simulink library "thc"  (R2021b)
settings: Solver=VariableStepAuto  StartTime=0.0  StopTime=10.0  RelTol=1e-3
undefined symbols (not defined in the file or in its folder): ATHC_ChargingPEUEWPReq_X_C, ATHC_ChargingPEUFanReq_X_C, ATHC_CoolingMCUEWPReq_X_C, ATHC_CoolingMCUFanReq_X_C, ATHC_CoolingPEUEWPReq_X_C, ATHC_CoolingPEUFanReq_X_C, ATHC_CoolingTMEWPReq_X_C, ATHC_CoolingTMFanReq_X_C, ENUM_ACCMODE_AFTERRUNNING, ENUM_ACCMODE_CHARGING, ENUM_ACCMODE_COOLING, ENUM_ACCMODE_OFF, ENUM_ACCMODE_SERVICE, ENUM_EWPPEFault_Running, ENUM_MCUFailGrade_NoFault, ENUM_PMMMODE_CHARGE, ENUM_PMMMODE_DRIVE, ENUM_PMMMODE_LVBATCHRG, ENUM_PMMMODE_POWERUP, KDSC_ServiceModeCoolFanReq_pct, KTHC_AfterrunMCUStartTemp_C, KTHC_AfterrunMCUStopTemp_C, KTHC_AfterrunningModeCoolFanReq_pct, KTHC_AfterrunningModeEWPPEReq_rpm, KTHC_AfterrunTMStartTemp_C, KTHC_AfterrunTMStopTemp_C, KTHC_CoolingEWPDisSpdDem_rpm, KTHC_CoolingEWPEnSpdDem_rpm, KTHC_CoolingFanPWMDis_pct, KTHC_CoolingFanPWMEn_pct, KTHC_EWPFaultBypassSwitch_flag, KTHC_EWPPEFaultSpd_rpm, KTHC_LostEWPCoolingFan_pct, KTHC_MCUDerationCoolFanReq_pct, KTHC_MCUDerationEWPPEReq_rpm, KTHC_MCUTempErrCoolFanReq_pct, KTHC_MCUTempErrEWPPEReq_rpm, KTHC_MCUTempError_C, KTHC_PEUDerationCoolFanReq_pct, KTHC_PEUDerationEWPPEReq_rpm, KTHC_PEUDerationTemp_C, KTHC_PEUTempErrCoolFanReq_pct, KTHC_PEUTempErrEWPPEReq_rpm, KTHC_PEUTempError_C, KTHC_ServiceModeCoolFanCMD_flg, KTHC_ServiceModeCoolFanReq_pct, KTHC_ServiceModeEWPPECMD_flg, KTHC_ServiceModeEWPPEReq_rpm, KTHC_ServiceModeON_flg, KTHC_TMTempErrCoolFanReq_pct, KTHC_TMTempErrEWPPEReq_rpm, KTHC_TMTempError_C, MTHC_ChargingPEUEWPReq_Y_rpm, MTHC_ChargingPEUFanReq_Y_pct, MTHC_CoolingMCUEWPReq_Y_rpm, MTHC_CoolingMCUFanReq_Y_pct, MTHC_CoolingPEUEWPReq_Y_rpm, MTHC_CoolingPEUFanReq_Y_pct, MTHC_CoolingTMEWPReq_Y_rpm, MTHC_CoolingTMFanReq_Y_pct ... (+2)
settings Model: Creator=FVT20341  LastModifiedBy=FVT22063

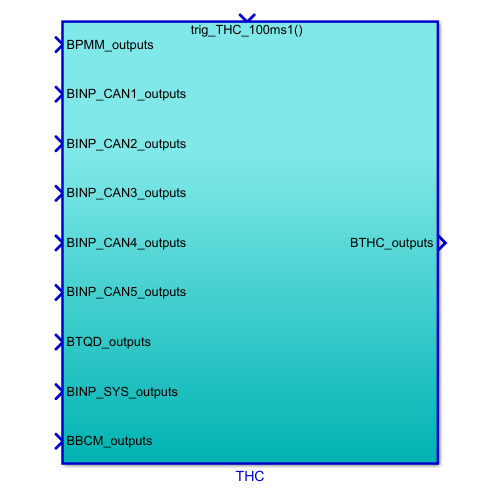
[thumbnail: Simulink's stored preview of the top-level diagram]
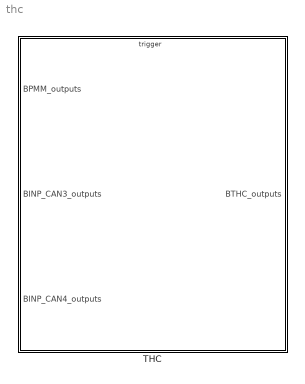
== system thc ==
  THC : Subsystem  TreatAsAtomicUnit=on
      settings: RTWSystemCode=Nonreusable function  RTWFcnNameOpts=Use subsystem name  RTWFileNameOpts=Use subsystem name

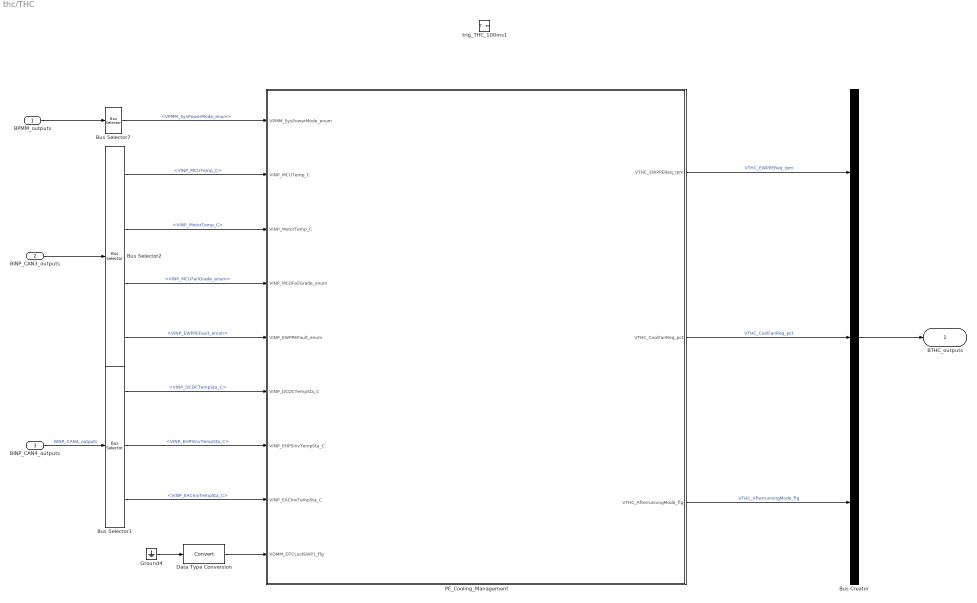
== system thc/THC ==
  BPMM_outputs : Inport  OutDataTypeStr=Bus: BPMM_outputs
  BINP_CAN3_outputs : Inport  Port=2  OutDataTypeStr=Bus: BINP_CAN3_outputs
  BINP_CAN4_outputs : Inport  Port=3  OutDataTypeStr=Bus: BINP_CAN4_outputs
  trig_THC_100ms1 : TriggerPort  TriggerType=function-call  VariantControl=(inherit)
  Bus Creator : BusCreator  Inputs=3  OutDataTypeStr=Bus: BTHC_outputs  NonVirtualBus=on
  Bus Selector1 : BusSelector  OutputSignals=VINP_DCDCTempSta_C,VINP_EHPSInvTempSta_C,VINP_EACInvTempSta_C
  Bus Selector2 : BusSelector  OutputSignals=VINP_MCUTemp_C,VINP_MotorTemp_C,VINP_MCUFailGrade_enum,VINP_EWPPEFault_enum
  Bus Selector7 : BusSelector  OutputSignals=VPMM_SysPowerMode_enum
  Data Type Conversion : DataTypeConversion
  Ground4 : Ground
  PE_Cooling_Management : Subsystem
  BTHC_outputs : Outport  OutDataTypeStr=Bus: BTHC_outputs
  wires:
  BPMM_outputs/1 -> Bus Selector7/1
  BINP_CAN3_outputs/1 -> Bus Selector2/1
  PE_Cooling_Management/1(VTHC_EWPPEReq_rpm) -> Bus Creator/1  "VTHC_EWPPEReq_rpm"
  PE_Cooling_Management/2(VTHC_CoolFanReq_pct) -> Bus Creator/2  "VTHC_CoolFanReq_pct"
  PE_Cooling_Management/3(VTHC_AfterrunningMode_flg) -> Bus Creator/3  "VTHC_AfterrunningMode_flg"
  Bus Creator/1 -> BTHC_outputs/1
  Bus Selector7/1 -> PE_Cooling_Management/1(VPMM_SysPowerMode_enum)  "<VPMM_SysPowerMode_enum>"
  Bus Selector2/1 -> PE_Cooling_Management/2(VINP_MCUTemp_C)  "<VINP_MCUTemp_C>"
  Bus Selector2/2 -> PE_Cooling_Management/3(VINP_MotorTemp_C)  "<VINP_MotorTemp_C>"
  Bus Selector2/3 -> PE_Cooling_Management/4(VINP_MCUFailGrade_enum)  "<VINP_MCUFailGrade_enum>"
  Bus Selector2/4 -> PE_Cooling_Management/5(VINP_EWPPEFault_enum)  "<VINP_EWPPEFault_enum>"
  BINP_CAN4_outputs/1 -> Bus Selector1/1  "BINP_CAN4_outputs"
  Bus Selector1/2 -> PE_Cooling_Management/7(VINP_EHPSInvTempSta_C)  "<VINP_EHPSInvTempSta_C>"
  Bus Selector1/1 -> PE_Cooling_Management/6(VINP_DCDCTempSta_C)  "<VINP_DCDCTempSta_C>"
  Bus Selector1/3 -> PE_Cooling_Management/8(VINP_EACInvTempSta_C)  "<VINP_EACInvTempSta_C>"
  Data Type Conversion/1 -> PE_Cooling_Management/9(VDMM_DTCLostEWP1_flg)
  Ground4/1 -> Data Type Conversion/1

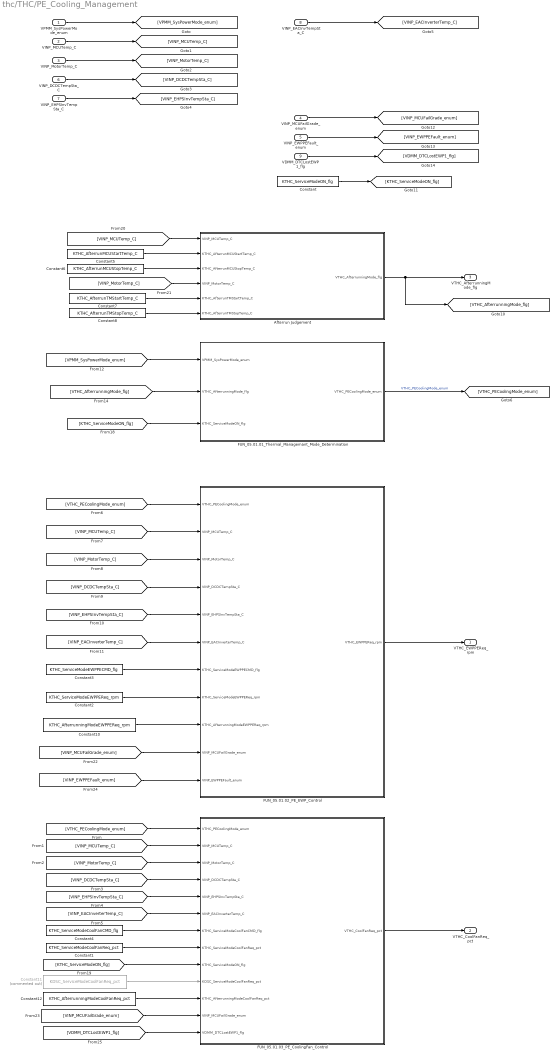
== system thc/THC/PE_Cooling_Management ==
  VPMM_SysPowerMode_enum : Inport
  VINP_MCUTemp_C : Inport  Port=2
  VINP_MotorTemp_C : Inport  Port=3
  VINP_MCUFailGrade_enum : Inport  Port=4
  VINP_EWPPEFault_enum : Inport  Port=5
  VINP_DCDCTempSta_C : Inport  Port=6
  VINP_EHPSInvTempSta_C : Inport  Port=7
  VINP_EACInvTempSta_C : Inport  Port=8
  VDMM_DTCLostEWP1_flg : Inport  Port=9
  Afterrun Judgement : Subsystem
  Constant : Constant  Value=KTHC_ServiceModeON_flg
  Constant1 : Constant  Value=KTHC_ServiceModeCoolFanReq_pct
  Constant10 : Constant  Value=KTHC_AfterrunningModeEWPPEReq_rpm
  Constant11 : Constant  Commented=on  Value=KDSC_ServiceModeCoolFanReq_pct
  Constant12 : Constant  Value=KTHC_AfterrunningModeCoolFanReq_pct
  Constant2 : Constant  Value=KTHC_ServiceModeEWPPEReq_rpm
  Constant3 : Constant  Value=KTHC_ServiceModeEWPPECMD_flg
  Constant4 : Constant  Value=KTHC_ServiceModeCoolFanCMD_flg
  Constant5 : Constant  Value=KTHC_AfterrunMCUStartTemp_C
  Constant6 : Constant  Value=KTHC_AfterrunMCUStopTemp_C
  Constant7 : Constant  Value=KTHC_AfterrunTMStartTemp_C
  Constant8 : Constant  Value=KTHC_AfterrunTMStopTemp_C
  FUN_05.01.01_Thermal_Managemant_Mode_Determination : Subsystem
  FUN_05.01.02_PE_EWP_Control : Subsystem
  FUN_05.01.03_PE_CoolingFan_Control : Subsystem
  VTHC_EWPPEReq_rpm : Outport
  VTHC_CoolFanReq_pct : Outport  Port=2
  VTHC_AfterrunningMode_flg : Outport  Port=3
  wires:
  [VTHC_AfterrunningMode_flg] -> FUN_05.01.01_Thermal_Managemant_Mode_Determination/2(VTHC_AfterrunningMode_flg)
  Constant2/1 -> FUN_05.01.02_PE_EWP_Control/8(KTHC_ServiceModeEWPPEReq_rpm)
  Constant3/1 -> FUN_05.01.02_PE_EWP_Control/7(KTHC_ServiceModeEWPPECMD_flg)
  [VINP_EACInverterTemp_C] -> FUN_05.01.02_PE_EWP_Control/6(VINP_EACInverterTemp_C)
  [VINP_EHPSInvTempSta_C] -> FUN_05.01.02_PE_EWP_Control/5(VINP_EHPSInvTempSta_C)
  [VINP_DCDCTempSta_C] -> FUN_05.01.02_PE_EWP_Control/4(VINP_DCDCTempSta_C)
  [VINP_MotorTemp_C] -> FUN_05.01.02_PE_EWP_Control/3(VINP_MotorTemp_C)
  [VINP_MCUTemp_C] -> FUN_05.01.02_PE_EWP_Control/2(VINP_MCUTemp_C)
  [VTHC_PECoolingMode_enum] -> FUN_05.01.02_PE_EWP_Control/1(VTHC_PECoolingMode_enum)
  Constant1/1 -> FUN_05.01.03_PE_CoolingFan_Control/8(KTHC_ServiceModeCoolFanReq_pct)
  Constant4/1 -> FUN_05.01.03_PE_CoolingFan_Control/7(KTHC_ServiceModeCoolFanCMD_flg)
  [VINP_EACInverterTemp_C] -> FUN_05.01.03_PE_CoolingFan_Control/6(VINP_EACInverterTemp_C)
  [VINP_EHPSInvTempSta_C] -> FUN_05.01.03_PE_CoolingFan_Control/5(VINP_EHPSInvTempSta_C)
  [VINP_DCDCTempSta_C] -> FUN_05.01.03_PE_CoolingFan_Control/4(VINP_DCDCTempSta_C)
  [VINP_MotorTemp_C] -> FUN_05.01.03_PE_CoolingFan_Control/3(VINP_MotorTemp_C)
  [VINP_MCUTemp_C] -> FUN_05.01.03_PE_CoolingFan_Control/2(VINP_MCUTemp_C)
  [VTHC_PECoolingMode_enum] -> FUN_05.01.03_PE_CoolingFan_Control/1(VTHC_PECoolingMode_enum)
  FUN_05.01.02_PE_EWP_Control/1(VTHC_EWPPEReq_rpm) -> VTHC_EWPPEReq_rpm/1
  FUN_05.01.03_PE_CoolingFan_Control/1(VTHC_CoolFanReq_pct) -> VTHC_CoolFanReq_pct/1
  [VPMM_SysPowerMode_enum] -> FUN_05.01.01_Thermal_Managemant_Mode_Determination/1(VPMM_SysPowerMode_enum)
  FUN_05.01.01_Thermal_Managemant_Mode_Determination/1(VTHC_PECoolingMode_enum) -> [VTHC_PECoolingMode_enum]  "VTHC_PECoolingMode_enum"
  VINP_MCUTemp_C/1 -> [VINP_MCUTemp_C]
  VINP_MotorTemp_C/1 -> [VINP_MotorTemp_C]
  VINP_DCDCTempSta_C/1 -> [VINP_DCDCTempSta_C]
  VINP_EHPSInvTempSta_C/1 -> [VINP_EHPSInvTempSta_C]
  VINP_EACInvTempSta_C/1 -> [VINP_EACInverterTemp_C]
  VPMM_SysPowerMode_enum/1 -> [VPMM_SysPowerMode_enum]
  Constant/1 -> [KTHC_ServiceModeON_flg]
  [KTHC_ServiceModeON_flg] -> FUN_05.01.01_Thermal_Managemant_Mode_Determination/3(KTHC_ServiceModeON_flg)
  [KTHC_ServiceModeON_flg] -> FUN_05.01.03_PE_CoolingFan_Control/9(KTHC_ServiceModeON_flg)
  Afterrun Judgement/1(VTHC_AfterrunningMode_flg) -> VTHC_AfterrunningMode_flg/1, [VTHC_AfterrunningMode_flg]
  [VINP_MotorTemp_C] -> Afterrun Judgement/4(VINP_MotorTemp_C)
  [VINP_MCUTemp_C] -> Afterrun Judgement/1(VINP_MCUTemp_C)
  Constant5/1 -> Afterrun Judgement/2(KTHC_AfterrunMCUStartTemp_C)
  Constant6/1 -> Afterrun Judgement/3(KTHC_AfterrunMCUStopTemp_C)
  Constant7/1 -> Afterrun Judgement/5(KTHC_AfterrunTMStartTemp_C)
  Constant8/1 -> Afterrun Judgement/6(KTHC_AfterrunTMStopTemp_C)
  Constant10/1 -> FUN_05.01.02_PE_EWP_Control/9(KTHC_AfterrunningModeEWPPEReq_rpm)
  Constant11/1 -> FUN_05.01.03_PE_CoolingFan_Control/10(KDSC_ServiceModeCoolFanReq_pct)
  Constant12/1 -> FUN_05.01.03_PE_CoolingFan_Control/11(KTHC_AfterrunningModeCoolFanReq_pct)
  VINP_MCUFailGrade_enum/1 -> [VINP_MCUFailGrade_enum]
  [VINP_MCUFailGrade_enum] -> FUN_05.01.02_PE_EWP_Control/10(VINP_MCUFailGrade_enum)
  [VINP_MCUFailGrade_enum] -> FUN_05.01.03_PE_CoolingFan_Control/12(VINP_MCUFailGrade_enum)
  VINP_EWPPEFault_enum/1 -> [VINP_EWPPEFault_enum]
  [VINP_EWPPEFault_enum] -> FUN_05.01.02_PE_EWP_Control/11(VINP_EWPPEFault_enum)
  VDMM_DTCLostEWP1_flg/1 -> [VDMM_DTCLostEWP1_flg]
  [VDMM_DTCLostEWP1_flg] -> FUN_05.01.03_PE_CoolingFan_Control/13(VDMM_DTCLostEWP1_flg)

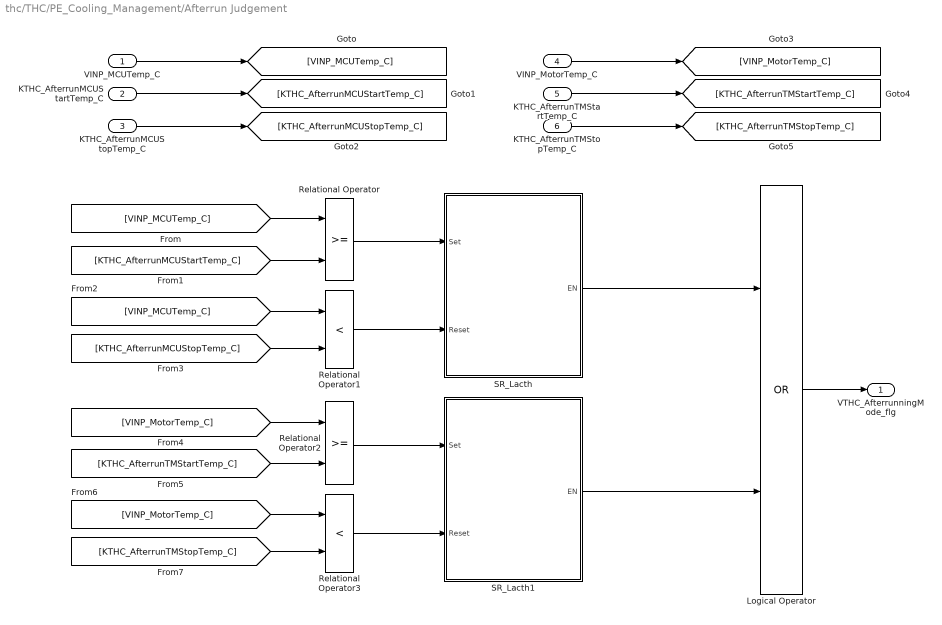
== system thc/THC/PE_Cooling_Management/Afterrun Judgement ==
  VINP_MCUTemp_C : Inport
  KTHC_AfterrunMCUStartTemp_C : Inport  Port=2
  KTHC_AfterrunMCUStopTemp_C : Inport  Port=3
  VINP_MotorTemp_C : Inport  Port=4
  KTHC_AfterrunTMStartTemp_C : Inport  Port=5
  KTHC_AfterrunTMStopTemp_C : Inport  Port=6
  Logical Operator : Logic  Operator=OR  AllPortsSameDT=off  OutDataTypeStr=boolean
  Relational Operator : RelationalOperator  OutDataTypeStr=boolean  RndMeth=Simplest
  Relational Operator1 : RelationalOperator  Operator=<  OutDataTypeStr=boolean  RndMeth=Simplest
  Relational Operator2 : RelationalOperator  OutDataTypeStr=boolean  RndMeth=Simplest
  Relational Operator3 : RelationalOperator  Operator=<  OutDataTypeStr=boolean  RndMeth=Simplest
  SR_Lacth : Subsystem
  SR_Lacth1 : Subsystem
  VTHC_AfterrunningMode_flg : Outport
  wires:
  SR_Lacth/1(EN) -> Logical Operator/1
  VINP_MCUTemp_C/1 -> [VINP_MCUTemp_C]
  KTHC_AfterrunMCUStartTemp_C/1 -> [KTHC_AfterrunMCUStartTemp_C]
  KTHC_AfterrunMCUStopTemp_C/1 -> [KTHC_AfterrunMCUStopTemp_C]
  VINP_MotorTemp_C/1 -> [VINP_MotorTemp_C]
  KTHC_AfterrunTMStartTemp_C/1 -> [KTHC_AfterrunTMStartTemp_C]
  KTHC_AfterrunTMStopTemp_C/1 -> [KTHC_AfterrunTMStopTemp_C]
  [VINP_MCUTemp_C] -> Relational Operator/1
  [KTHC_AfterrunMCUStartTemp_C] -> Relational Operator/2
  Relational Operator/1 -> SR_Lacth/1(Set)
  [KTHC_AfterrunMCUStopTemp_C] -> Relational Operator1/2
  [VINP_MCUTemp_C] -> Relational Operator1/1
  Relational Operator1/1 -> SR_Lacth/2(Reset)
  [KTHC_AfterrunTMStopTemp_C] -> Relational Operator3/2
  [VINP_MotorTemp_C] -> Relational Operator2/1
  SR_Lacth1/1(EN) -> Logical Operator/2
  [KTHC_AfterrunTMStartTemp_C] -> Relational Operator2/2
  Relational Operator3/1 -> SR_Lacth1/2(Reset)
  [VINP_MotorTemp_C] -> Relational Operator3/1
  Logical Operator/1 -> VTHC_AfterrunningMode_flg/1
  Relational Operator2/1 -> SR_Lacth1/1(Set)

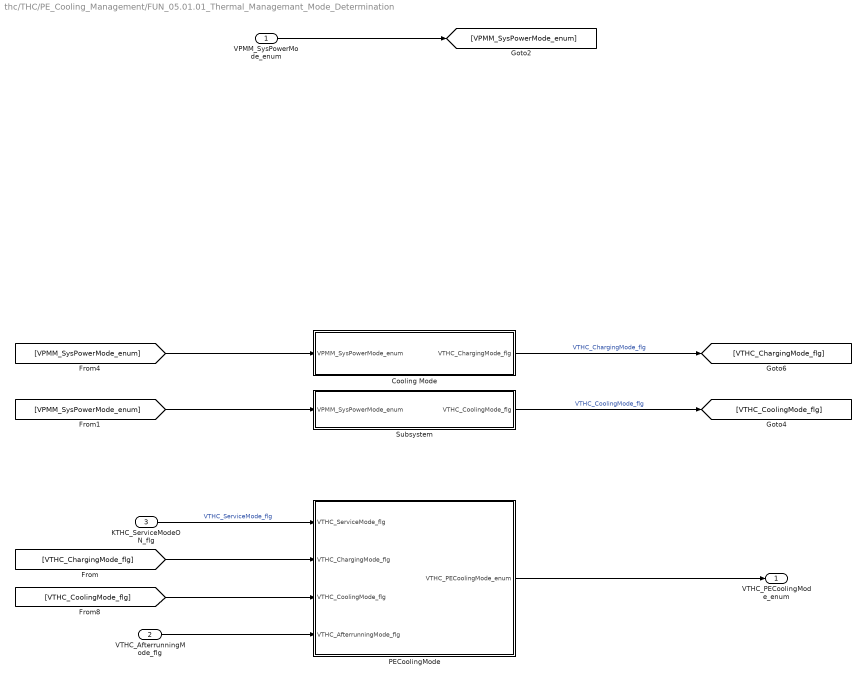
== system thc/THC/PE_Cooling_Management/FUN_05.01.01_Thermal_Managemant_Mode_Determination ==
  VPMM_SysPowerMode_enum : Inport
  VTHC_AfterrunningMode_flg : Inport  Port=2
  KTHC_ServiceModeON_flg : Inport  Port=3
  Cooling Mode : Subsystem
  PECoolingMode : Subsystem
  Subsystem : Subsystem
  VTHC_PECoolingMode_enum : Outport  VectorParamsAs1DForOutWhenUnconnected=off
  wires:
  VTHC_AfterrunningMode_flg/1 -> PECoolingMode/4(VTHC_AfterrunningMode_flg)
  [VTHC_CoolingMode_flg] -> PECoolingMode/3(VTHC_CoolingMode_flg)
  [VTHC_ChargingMode_flg] -> PECoolingMode/2(VTHC_ChargingMode_flg)
  KTHC_ServiceModeON_flg/1 -> PECoolingMode/1(VTHC_ServiceMode_flg)  "VTHC_ServiceMode_flg"
  [VPMM_SysPowerMode_enum] -> Subsystem/1(VPMM_SysPowerMode_enum)
  Subsystem/1(VTHC_CoolingMode_flg) -> [VTHC_CoolingMode_flg]  "VTHC_CoolingMode_flg"
  PECoolingMode/1(VTHC_PECoolingMode_enum) -> VTHC_PECoolingMode_enum/1
  [VPMM_SysPowerMode_enum] -> Cooling Mode/1(VPMM_SysPowerMode_enum)
  VPMM_SysPowerMode_enum/1 -> [VPMM_SysPowerMode_enum]
  Cooling Mode/1(VTHC_ChargingMode_flg) -> [VTHC_ChargingMode_flg]  "VTHC_ChargingMode_flg"

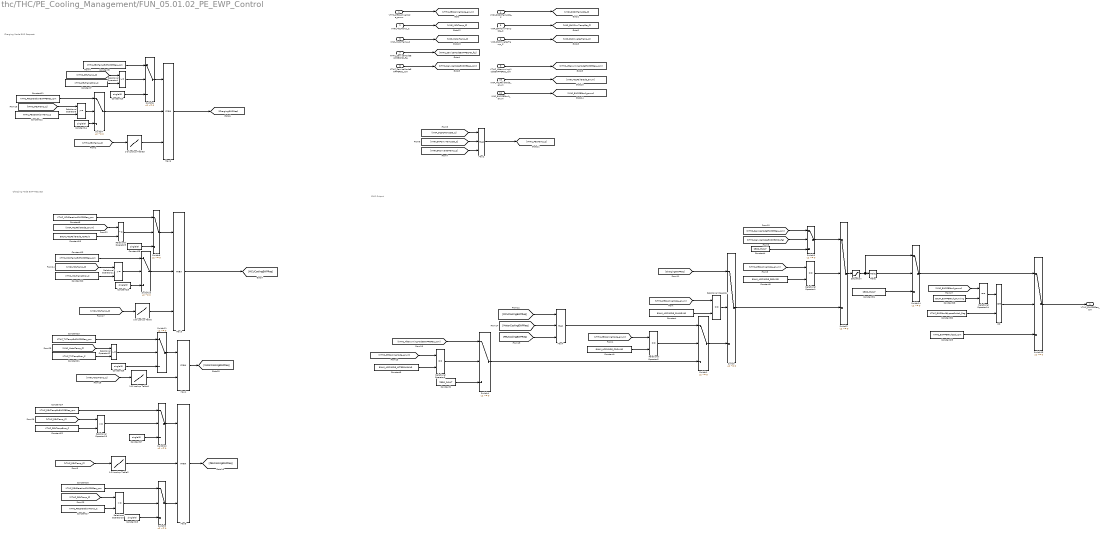
== system thc/THC/PE_Cooling_Management/FUN_05.01.02_PE_EWP_Control ==
  note: EWP Output
  note: Charging Mode EWP Request
  note: Charging Mode EWP Request
  VTHC_PECoolingMode_enum : Inport
  VINP_MCUTemp_C : Inport  Port=2
  VINP_MotorTemp_C : Inport  Port=3
  VINP_DCDCTempSta_C : Inport  Port=4
  VINP_EHPSInvTempSta_C : Inport  Port=5
  VINP_EACInverterTemp_C : Inport  Port=6
  KTHC_ServiceModeEWPPECMD_flg : Inport  Port=7
  KTHC_ServiceModeEWPPEReq_rpm : Inport  Port=8
  KTHC_AfterrunningModeEWPPEReq_rpm : Inport  Port=9
  VINP_MCUFailGrade_enum : Inport  Port=10
  VINP_EWPPEFault_enum : Inport  Port=11
  1-D Lookup Table : Lookup_n-D  NumberOfTableDimensions=1  BreakpointsForDimension1=ATHC_CoolingMCUEWPReq_X_C  Table=MTHC_CoolingMCUEWPReq_Y_rpm  ExtrapMethod=Clip  UseLastTableValue=on  InternalRulePriority=Speed  RndMeth=Simplest  InputSameDT=on
  1-D Lookup Table1 : Lookup_n-D  NumberOfTableDimensions=1  BreakpointsForDimension1=ATHC_CoolingTMEWPReq_X_C  Table=MTHC_CoolingTMEWPReq_Y_rpm  ExtrapMethod=Clip  UseLastTableValue=on  InternalRulePriority=Speed  RndMeth=Simplest  InputSameDT=on
  1-D Lookup Table2 : Lookup_n-D  NumberOfTableDimensions=1  BreakpointsForDimension1=ATHC_CoolingPEUEWPReq_X_C  Table=MTHC_CoolingPEUEWPReq_Y_rpm  ExtrapMethod=Clip  UseLastTableValue=on  InternalRulePriority=Speed  RndMeth=Simplest  InputSameDT=on
  1-D Lookup Table3 : Lookup_n-D  NumberOfTableDimensions=1  BreakpointsForDimension1=ATHC_ChargingPEUEWPReq_X_C  Table=MTHC_ChargingPEUEWPReq_Y_rpm  ExtrapMethod=Clip  UseLastTableValue=on  InternalRulePriority=Speed  RndMeth=Simplest  InputSameDT=on
  Constant : Constant  Value=ENUM_ACCMODE_CHARGING
  Constant1 : Constant  Value=ENUM_ACCMODE_COOLING
  Constant{10,14,18..19,25..27} (7 alike) : Constant  Value=single(0)
  Constant11 : Constant  Value=KTHC_PEUDerationEWPPEReq_rpm
  Constant12 : Constant  Value=KTHC_PEUDerationTemp_C
  Constant13 : Constant  Value=KTHC_MCUTempErrEWPPEReq_rpm
  Constant15 : Constant  Value=ENUM_MCUFailGrade_NoFault
  Constant16 : Constant  Value=KTHC_PEUDerationEWPPEReq_rpm
  Constant17 : Constant  Value=KTHC_PEUDerationTemp_C
  Constant2 : Constant  Value=ZERO_FLOAT
  Constant20 : Constant  Value=KTHC_MCUTempError_C
  Constant21 : Constant  Value=KTHC_TMTempError_C
  Constant22 : Constant  Value=KTHC_PEUTempError_C
  Constant23 : Constant  Value=KTHC_TMTempErrEWPPEReq_rpm
  Constant24 : Constant  Value=KTHC_PEUTempErrEWPPEReq_rpm
  Constant28 : Constant  Value=ENUM_EWPPEFault_Running
  Constant29 : Constant  Value=KTHC_EWPPEFaultSpd_rpm
  Constant3 : Constant  Value=ENUM_ACCMODE_SERVICE
  Constant30 : Constant  Value=KTHC_EWPFaultBypassSwitch_flag  VectorParams1D=off
  Constant31 : Constant  Value=ZERO_FLOAT
  Constant4 : Constant  Value=ZERO_FLOAT
  Constant5 : Constant  Value=ENUM_ACCMODE_AFTERRUNNING
  Constant7 : Constant  Value=KTHC_PEUTempError_C
  Constant8 : Constant  Value=KTHC_MCUDerationEWPPEReq_rpm
  Constant9 : Constant  Value=KTHC_PEUTempErrEWPPEReq_rpm
  Max1 : MinMax  Function=max  Inputs=2
  Max{2..6} (5 alike) : MinMax  Function=max  Inputs=3
  OR : Logic  Operator=OR  AllPortsSameDT=off  OutDataTypeStr=boolean
  Relational Operator{,1..3,14} (5 alike) : RelationalOperator  Operator===  OutDataTypeStr=boolean  RndMeth=Simplest
  Relational Operator{4..5,10..13} (6 alike) : RelationalOperator  OutDataTypeStr=boolean  RndMeth=Simplest
  Relational Operator9 : RelationalOperator  Operator=~=  OutDataTypeStr=boolean  RndMeth=Simplest
  Relay : Relay  OnSwitchValue=KTHC_CoolingEWPEnSpdDem_rpm  OffSwitchValue=KTHC_CoolingEWPDisSpdDem_rpm  OnOutputValue=TRUE  OffOutputValue=FALSE  OutDataTypeStr=boolean
  Saturation : Saturate  UpperLimit=6000  LowerLimit=0
  Switch{,1..4,6..14} (14 alike) : Switch  Criteria=u2 ~= 0
  VTHC_EWPPEReq_rpm : Outport
  wires:
  VINP_MCUTemp_C/1 -> [VINP_MCUTemp_C]
  Switch2/1 -> Saturation/1
  [KTHC_AfterrunningModeEWPPEReq_rpm] -> Switch4/1
  Constant2/1 -> Switch4/3
  [VTHC_PECoolingMode_enum] -> Relational Operator3/1
  Relational Operator3/1 -> Switch4/2
  Constant5/1 -> Relational Operator3/2
  Switch4/1 -> Switch1/3
  KTHC_ServiceModeEWPPEReq_rpm/1 -> [KTHC_ServiceModeEWPPEReq_rpm]
  KTHC_ServiceModeEWPPECMD_flg/1 -> [KTHC_ServiceModeEWPPECMD_flg]
  VINP_MotorTemp_C/1 -> [VINP_MotorTemp_C]
  VTHC_PECoolingMode_enum/1 -> [VTHC_PECoolingMode_enum]
  [VTHC_PECoolingMode_enum] -> Relational Operator/1
  [VTHC_PECoolingMode_enum] -> Relational Operator2/1
  [VINP_EACInverterTemp_C] -> Max2/3
  [VINP_DCDCTempSta_C] -> Max2/1
  [VINP_EHPSInvTempSta_C] -> Max2/2
  Relational Operator/1 -> Switch/2
  Max2/1 -> [VTHC_PEUTemp_C]
  [VTHC_PEUTemp_C] -> 1-D Lookup Table2/1
  Constant1/1 -> Relational Operator2/2
  [KTHC_ServiceModeEWPPECMD_flg] -> Switch3/2
  Switch/1 -> Switch2/3
  Constant/1 -> Relational Operator/2
  Switch1/1 -> Switch/3
  Relational Operator2/1 -> Switch1/2
  Relational Operator1/1 -> Switch2/2
  Constant4/1 -> Switch3/3
  [VTHC_PECoolingMode_enum] -> Relational Operator1/1
  Constant3/1 -> Relational Operator1/2
  [KTHC_ServiceModeEWPPEReq_rpm] -> Switch3/1
  VINP_DCDCTempSta_C/1 -> [VINP_DCDCTempSta_C]
  VINP_EHPSInvTempSta_C/1 -> [VINP_EHPSInvTempSta_C]
  VINP_EACInverterTemp_C/1 -> [VINP_EACInverterTemp_C]
  Switch3/1 -> Switch2/1
  KTHC_AfterrunningModeEWPPEReq_rpm/1 -> [KTHC_AfterrunningModeEWPPEReq_rpm]
  VINP_MCUFailGrade_enum/1 -> [VINP_MCUFailGrade_enum]
  [VTHC_PEUTemp_C] -> 1-D Lookup Table3/1
  [VINP_MCUTemp_C] -> 1-D Lookup Table/1
  [VINP_MotorTemp_C] -> 1-D Lookup Table1/1
  [VINP_MCUFailGrade_enum] -> Relational Operator9/1
  Relational Operator9/1 -> Switch8/2
  Constant15/1 -> Relational Operator9/2
  Constant16/1 -> Switch9/1
  Constant17/1 -> Relational Operator10/2
  Relational Operator10/1 -> Switch9/2
  [VTHC_PEUTemp_C] -> Relational Operator10/1
  Constant8/1 -> Switch8/1
  Constant18/1 -> Switch8/3
  Constant19/1 -> Switch9/3
  Constant20/1 -> Relational Operator11/2
  Constant22/1 -> Relational Operator13/2
  [VINP_MCUTemp_C] -> Relational Operator11/1
  [VINP_MotorTemp_C] -> Relational Operator12/1
  [VTHC_PEUTemp_C] -> Relational Operator13/1
  Constant21/1 -> Relational Operator12/2
  Relational Operator11/1 -> Switch10/2
  Relational Operator12/1 -> Switch11/2
  Relational Operator13/1 -> Switch12/2
  Constant25/1 -> Switch10/3
  Constant26/1 -> Switch11/3
  Constant27/1 -> Switch12/3
  Constant24/1 -> Switch12/1
  Constant23/1 -> Switch11/1
  Constant13/1 -> Switch10/1
  VINP_EWPPEFault_enum/1 -> [VINP_EWPPEFault_enum]
  [VINP_EWPPEFault_enum] -> Relational Operator14/1
  Constant28/1 -> Relational Operator14/2
  Switch13/1 -> VTHC_EWPPEReq_rpm/1
  Constant29/1 -> Switch13/3
  Switch10/1 -> Max3/2
  1-D Lookup Table/1 -> Max3/3
  Switch8/1 -> Max3/1
  Switch11/1 -> Max1/1
  1-D Lookup Table1/1 -> Max1/2
  Switch12/1 -> Max5/1
  1-D Lookup Table2/1 -> Max5/2
  Switch9/1 -> Max5/3
  Max3/1 -> [MCUCoolingEWPReq]
  [VTHC_PEUTemp_C] -> Relational Operator4/1
  Relational Operator4/1 -> Switch6/2
  Constant12/1 -> Relational Operator5/2
  Constant9/1 -> Switch6/1
  Constant7/1 -> Relational Operator4/2
  Constant11/1 -> Switch7/1
  Relational Operator5/1 -> Switch7/2
  Constant10/1 -> Switch6/3
  [VTHC_PEUTemp_C] -> Relational Operator5/1
  Constant14/1 -> Switch7/3
  Switch6/1 -> Max6/1
  Switch7/1 -> Max6/2
  1-D Lookup Table3/1 -> Max6/3
  Max6/1 -> [ChargingEWPReq]
  Relational Operator14/1 -> OR/1
  Saturation/1 -> Relay/1, Switch14/1  "VTHC_OriginalEWPSpdDem_rpm"
  Relay/1 -> Switch14/2  "VTHC_EWPSpdDemRelay_flg"
  Switch14/1 -> Switch13/1
  Constant31/1 -> Switch14/3
  Constant30/1 -> OR/2
  OR/1 -> Switch13/2
  [ChargingEWPReq] -> Switch/1
  Max1/1 -> [MotorCoolingEWPReq]
  Max5/1 -> [PEUCoolingEWPReq]
  Max4/1 -> Switch1/1
  [MCUCoolingEWPReq] -> Max4/1
  [MotorCoolingEWPReq] -> Max4/2
  [PEUCoolingEWPReq] -> Max4/3

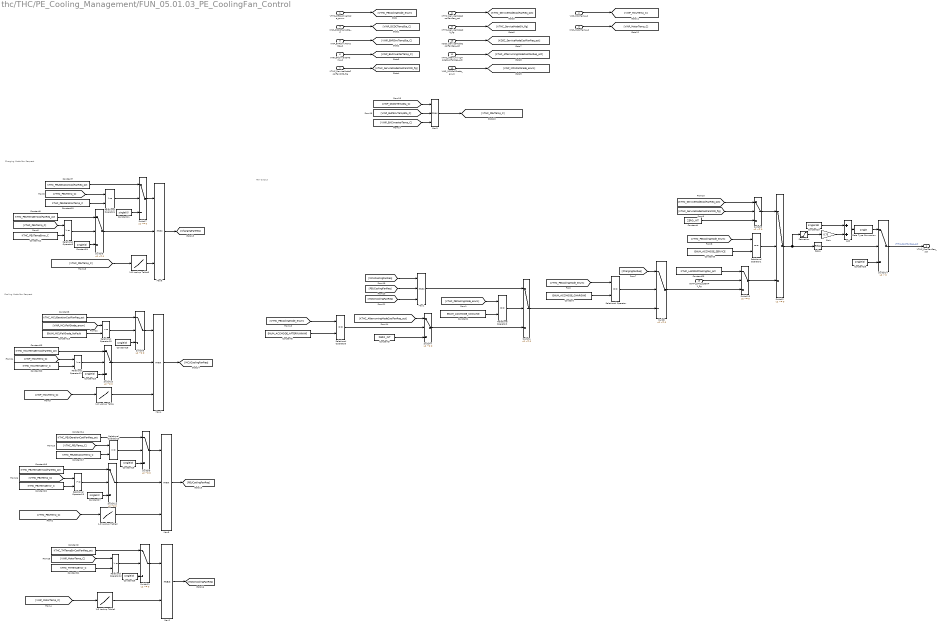
== system thc/THC/PE_Cooling_Management/FUN_05.01.03_PE_CoolingFan_Control ==
  note: Fan Output
  note: Cooling Mode Fan Request
  note: Charging Mode Fan Request
  VTHC_PECoolingMode_enum : Inport
  VINP_MCUTemp_C : Inport  Port=2
  VINP_MotorTemp_C : Inport  Port=3
  VINP_DCDCTempSta_C : Inport  Port=4
  VINP_EHPSInvTempSta_C : Inport  Port=5
  VINP_EACInverterTemp_C : Inport  Port=6
  KTHC_ServiceModeCoolFanCMD_flg : Inport  Port=7
  KTHC_ServiceModeCoolFanReq_pct : Inport  Port=8
  KTHC_ServiceModeON_flg : Inport  Port=9
  KDSC_ServiceModeCoolFanReq_pct : Inport  Port=10
  KTHC_AfterrunningModeCoolFanReq_pct : Inport  Port=11
  VINP_MCUFailGrade_enum : Inport  Port=12
  VDMM_DTCLostEWP1_flg : Inport  Port=13
  1-D Lookup Table : Lookup_n-D  NumberOfTableDimensions=1  BreakpointsForDimension1=ATHC_CoolingMCUFanReq_X_C  Table=MTHC_CoolingMCUFanReq_Y_pct  ExtrapMethod=Clip  UseLastTableValue=on  InternalRulePriority=Speed  RndMeth=Simplest  InputSameDT=on
  1-D Lookup Table1 : Lookup_n-D  NumberOfTableDimensions=1  BreakpointsForDimension1=ATHC_CoolingTMFanReq_X_C  Table=MTHC_CoolingTMFanReq_Y_pct  ExtrapMethod=Clip  UseLastTableValue=on  InternalRulePriority=Speed  RndMeth=Simplest  InputSameDT=on
  1-D Lookup Table2 : Lookup_n-D  NumberOfTableDimensions=1  BreakpointsForDimension1=ATHC_CoolingPEUFanReq_X_C  Table=MTHC_CoolingPEUFanReq_Y_pct  ExtrapMethod=Clip  UseLastTableValue=on  InternalRulePriority=Speed  RndMeth=Simplest  InputSameDT=on
  1-D Lookup Table3 : Lookup_n-D  NumberOfTableDimensions=1  BreakpointsForDimension1=ATHC_ChargingPEUFanReq_X_C  Table=MTHC_ChargingPEUFanReq_Y_pct  ExtrapMethod=Clip  UseLastTableValue=on  InternalRulePriority=Speed  RndMeth=Simplest  InputSameDT=on
  Add : Sum
  Constant : Constant  Value=ENUM_ACCMODE_CHARGING
  Constant1 : Constant  Value=ENUM_ACCMODE_COOLING
  Constant10 : Constant  Value=KTHC_PEUDerationTemp_C
  Constant{11,18..19,24..28} (8 alike) : Constant  Value=single(0)
  Constant12 : Constant  Value=KTHC_PEUTempError_C
  Constant13 : Constant  Value=KTHC_MCUTempErrCoolFanReq_pct
  Constant14 : Constant  Value=KTHC_PEUDerationCoolFanReq_pct
  Constant15 : Constant  Value=ENUM_MCUFailGrade_NoFault
  Constant16 : Constant  Value=KTHC_PEUTempErrCoolFanReq_pct
  Constant17 : Constant  Value=KTHC_PEUDerationTemp_C
  Constant2 : Constant  Value=KTHC_TMTempErrCoolFanReq_pct
  Constant20 : Constant  Value=KTHC_MCUTempError_C
  Constant21 : Constant  Value=KTHC_TMTempError_C
  Constant22 : Constant  Value=KTHC_PEUTempError_C
  Constant23 : Constant  Value=KTHC_LostEWPCoolingFan_pct
  Constant29 : Constant  Value=single(15)
  Constant3 : Constant  Value=ENUM_ACCMODE_SERVICE
  Constant4 : Constant  Value=ZERO_INT
  Constant5 : Constant  Value=ZERO_INT
  Constant6 : Constant  Value=ENUM_ACCMODE_AFTERRUNNING
  Constant7 : Constant  Value=KTHC_PEUDerationCoolFanReq_pct
  Constant8 : Constant  Value=KTHC_MCUDerationCoolFanReq_pct
  Constant9 : Constant  Value=KTHC_PEUTempErrCoolFanReq_pct
  Data Type Conversion : DataTypeConversion  OutDataTypeStr=single
  Gain : Gain  Gain=0.75
  Max{1,3..6} (5 alike) : MinMax  Function=max  Inputs=3
  Max2 : MinMax  Function=max  Inputs=2
  Relational Operator{,1..3} (4 alike) : RelationalOperator  Operator===  OutDataTypeStr=boolean  RndMeth=Simplest
  Relational Operator{4..5,10..13} (6 alike) : RelationalOperator  OutDataTypeStr=boolean  RndMeth=Simplest
  Relational Operator15 : RelationalOperator  Operator=~=  OutDataTypeStr=boolean  RndMeth=Simplest
  Relay : Relay  OnSwitchValue=KTHC_CoolingFanPWMEn_pct  OffSwitchValue=KTHC_CoolingFanPWMDis_pct  OnOutputValue=TRUE  OffOutputValue=FALSE  OutDataTypeStr=boolean
  Saturation : Saturate  UpperLimit=100  LowerLimit=0
  Switch{,1..4,6..13} (13 alike) : Switch  Criteria=u2 ~= 0
  Switch14 : Switch  Criteria=u2 > Threshold
  VTHC_CoolFanReq_pct : Outport
  wires:
  Switch14/1 -> VTHC_CoolFanReq_pct/1  "VTHC_CoolFanReq_pct"
  Switch4/1 -> Switch1/3
  Constant5/1 -> Switch4/3
  [KTHC_AfterrunningModeCoolFanReq_pct] -> Switch4/1
  Constant6/1 -> Relational Operator3/2
  [VTHC_PECoolingMode_enum] -> Relational Operator3/1
  Relational Operator3/1 -> Switch4/2
  Constant4/1 -> Switch3/3
  [KTHC_ServiceModeCoolFanCMD_flg] -> Switch3/2
  [KTHC_ServiceModeCoolFanReq_pct] -> Switch3/1
  KTHC_ServiceModeCoolFanCMD_flg/1 -> [KTHC_ServiceModeCoolFanCMD_flg]
  KTHC_ServiceModeCoolFanReq_pct/1 -> [KTHC_ServiceModeCoolFanReq_pct]
  [VTHC_PECoolingMode_enum] -> Relational Operator1/1
  Relational Operator1/1 -> Switch2/2
  Constant3/1 -> Relational Operator1/2
  [VTHC_PEUTemp_C] -> 1-D Lookup Table3/1
  VINP_EACInverterTemp_C/1 -> [VINP_EACInverterTemp_C]
  VINP_EHPSInvTempSta_C/1 -> [VINP_EHPSInvTempSta_C]
  VINP_DCDCTempSta_C/1 -> [VINP_DCDCTempSta_C]
  [VTHC_PEUTemp_C] -> 1-D Lookup Table2/1
  VINP_MotorTemp_C/1 -> [VINP_MotorTemp_C]
  VINP_MCUTemp_C/1 -> [VINP_MCUTemp_C]
  Switch1/1 -> Switch/3
  Relational Operator2/1 -> Switch1/2
  Relational Operator/1 -> Switch/2
  Constant1/1 -> Relational Operator2/2
  [VTHC_PECoolingMode_enum] -> Relational Operator2/1
  [VTHC_PECoolingMode_enum] -> Relational Operator/1
  VTHC_PECoolingMode_enum/1 -> [VTHC_PECoolingMode_enum]
  Constant/1 -> Relational Operator/2
  KTHC_ServiceModeON_flg/1 -> [KTHC_ServiceModeON_flg]
  Switch3/1 -> Switch2/1
  KDSC_ServiceModeCoolFanReq_pct/1 -> [KDSC_ServiceModeCoolFanReq_pct]
  KTHC_AfterrunningModeCoolFanReq_pct/1 -> [KTHC_AfterrunningModeCoolFanReq_pct]
  VINP_MCUFailGrade_enum/1 -> [VINP_MCUFailGrade_enum]
  [VINP_EHPSInvTempSta_C] -> Max3/2
  [VINP_DCDCTempSta_C] -> Max3/1
  [VINP_EACInverterTemp_C] -> Max3/3
  Max3/1 -> [VTHC_PEUTemp_C]
  [VINP_MCUTemp_C] -> 1-D Lookup Table/1
  [VINP_MotorTemp_C] -> 1-D Lookup Table1/1
  [VTHC_PEUTemp_C] -> Relational Operator10/1
  Relational Operator15/1 -> Switch8/2
  [VINP_MCUTemp_C] -> Relational Operator11/1
  Constant22/1 -> Relational Operator13/2
  Constant21/1 -> Relational Operator12/2
  [VTHC_PEUTemp_C] -> Relational Operator13/1
  [VINP_MotorTemp_C] -> Relational Operator12/1
  Constant16/1 -> Switch12/1
  Relational Operator13/1 -> Switch12/2
  Constant15/1 -> Relational Operator15/2
  [VINP_MCUFailGrade_enum] -> Relational Operator15/1
  Constant14/1 -> Switch9/1
  Relational Operator10/1 -> Switch9/2
  Constant25/1 -> Switch10/3
  Constant2/1 -> Switch11/1
  Constant26/1 -> Switch11/3
  Relational Operator12/1 -> Switch11/2
  Constant17/1 -> Relational Operator10/2
  Relational Operator11/1 -> Switch10/2
  Constant19/1 -> Switch9/3
  Constant27/1 -> Switch12/3
  Constant20/1 -> Relational Operator11/2
  Constant18/1 -> Switch8/3
  Constant13/1 -> Switch10/1
  Constant8/1 -> Switch8/1
  Switch/1 -> Switch13/3
  Switch13/1 -> Switch2/3
  VDMM_DTCLostEWP1_flg/1 -> Switch13/2
  Constant23/1 -> Switch13/1
  Switch8/1 -> Max4/1
  Switch10/1 -> Max4/2
  1-D Lookup Table/1 -> Max4/3
  Switch9/1 -> Max5/1
  Switch12/1 -> Max5/2
  1-D Lookup Table2/1 -> Max5/3
  Switch11/1 -> Max2/1
  1-D Lookup Table1/1 -> Max2/2
  Max1/1 -> Switch1/1
  [VTHC_PEUTemp_C] -> Relational Operator5/1
  Constant12/1 -> Relational Operator5/2
  Constant11/1 -> Switch7/3
  Relational Operator4/1 -> Switch7/2
  Constant7/1 -> Switch7/1
  Constant10/1 -> Relational Operator4/2
  [VTHC_PEUTemp_C] -> Relational Operator4/1
  Constant24/1 -> Switch6/3
  Constant9/1 -> Switch6/1
  Relational Operator5/1 -> Switch6/2
  Switch7/1 -> Max6/1
  Switch6/1 -> Max6/2
  1-D Lookup Table3/1 -> Max6/3
  Relay/1 -> Switch14/2
  Switch2/1 -> Saturation/1, Relay/1
  Constant28/1 -> Switch14/3
  Max6/1 -> [ChargingFanReq]
  [ChargingFanReq] -> Switch/1
  Max4/1 -> [MCUCoolingFanReq]
  [MCUCoolingFanReq] -> Max1/1
  Max5/1 -> [PEUCoolingFanReq]
  Max2/1 -> [MotorCoolingFanReq]
  [MotorCoolingFanReq] -> Max1/3
  [PEUCoolingFanReq] -> Max1/2
  Saturation/1 -> Gain/1
  Gain/1 -> Add/2
  Constant29/1 -> Add/1
  Add/1 -> Data Type Conversion/1
  Data Type Conversion/1 -> Switch14/1

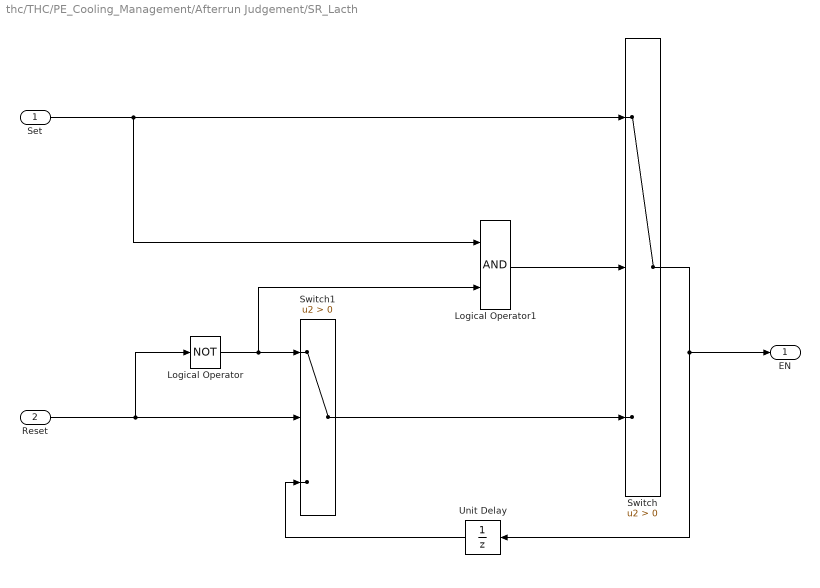
== system thc/THC/PE_Cooling_Management/Afterrun Judgement/SR_Lacth ==
  Set : Inport
  Reset : Inport  Port=2
  Logical Operator : Logic  Operator=NOT  AllPortsSameDT=off  OutDataTypeStr=boolean
  Logical Operator1 : Logic  AllPortsSameDT=off  OutDataTypeStr=boolean
  Switch : Switch  Criteria=u2 > Threshold
  Switch1 : Switch  Criteria=u2 > Threshold
  Unit Delay : UnitDelay  SampleTime=-1  HasFrameUpgradeWarning=on
  EN : Outport
  wires:
  Switch1/1 -> Switch/3
  Unit Delay/1 -> Switch1/3
  Logical Operator/1 -> Logical Operator1/2, Switch1/1
  Set/1 -> Logical Operator1/1, Switch/1
  Switch/1 -> EN/1, Unit Delay/1
  Reset/1 -> Logical Operator/1, Switch1/2
  Logical Operator1/1 -> Switch/2

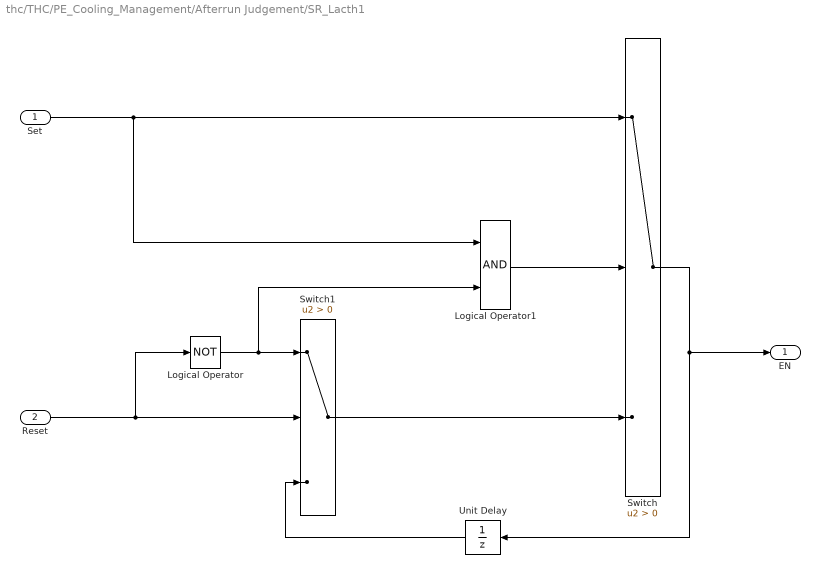
== system thc/THC/PE_Cooling_Management/Afterrun Judgement/SR_Lacth1 ==
  Set : Inport
  Reset : Inport  Port=2
  Logical Operator : Logic  Operator=NOT  AllPortsSameDT=off  OutDataTypeStr=boolean
  Logical Operator1 : Logic  AllPortsSameDT=off  OutDataTypeStr=boolean
  Switch : Switch  Criteria=u2 > Threshold
  Switch1 : Switch  Criteria=u2 > Threshold
  Unit Delay : UnitDelay  SampleTime=-1  HasFrameUpgradeWarning=on
  EN : Outport
  wires:
  Logical Operator1/1 -> Switch/2
  Reset/1 -> Switch1/2, Logical Operator/1
  Switch/1 -> Unit Delay/1, EN/1
  Set/1 -> Switch/1, Logical Operator1/1
  Logical Operator/1 -> Switch1/1, Logical Operator1/2
  Unit Delay/1 -> Switch1/3
  Switch1/1 -> Switch/3

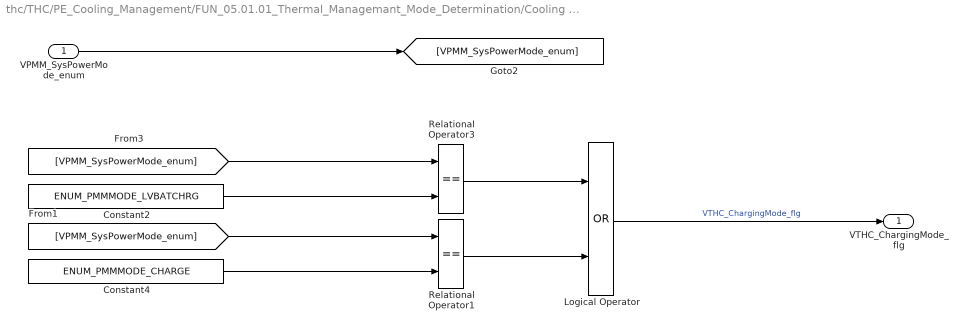
== system thc/THC/PE_Cooling_Management/FUN_05.01.01_Thermal_Managemant_Mode_Determination/Cooling Mode ==
  VPMM_SysPowerMode_enum : Inport
  Constant2 : Constant  Value=ENUM_PMMMODE_LVBATCHRG  SampleTime=-1
  Constant4 : Constant  Value=ENUM_PMMMODE_CHARGE  SampleTime=-1
  Logical Operator : Logic  Operator=OR  AllPortsSameDT=off  OutDataTypeStr=boolean
  Relational Operator1 : RelationalOperator  Operator===  OutDataTypeStr=boolean  RndMeth=Nearest
  Relational Operator3 : RelationalOperator  Operator===  OutDataTypeStr=boolean  RndMeth=Nearest
  VTHC_ChargingMode_flg : Outport  VectorParamsAs1DForOutWhenUnconnected=off
  wires:
  [VPMM_SysPowerMode_enum] -> Relational Operator3/1
  Constant2/1 -> Relational Operator3/2
  VPMM_SysPowerMode_enum/1 -> [VPMM_SysPowerMode_enum]
  [VPMM_SysPowerMode_enum] -> Relational Operator1/1
  Constant4/1 -> Relational Operator1/2
  Relational Operator3/1 -> Logical Operator/1
  Relational Operator1/1 -> Logical Operator/2
  Logical Operator/1 -> VTHC_ChargingMode_flg/1  "VTHC_ChargingMode_flg"

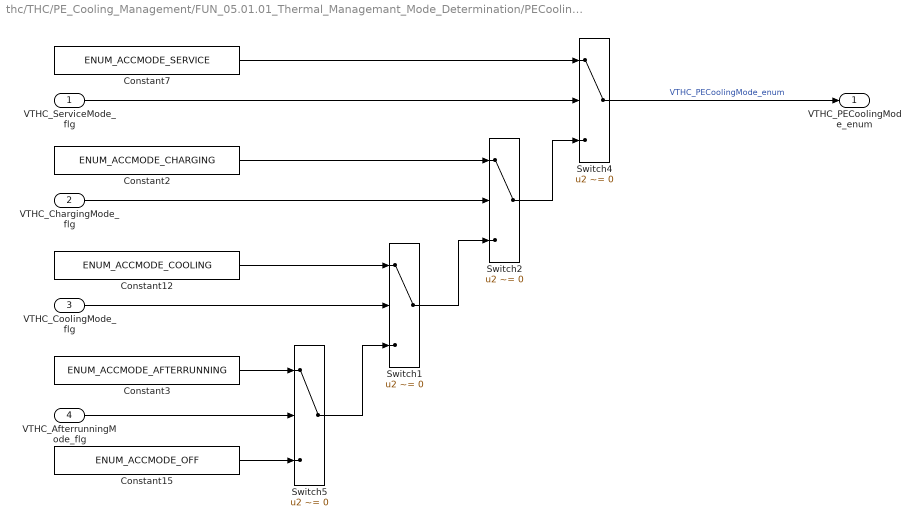
== system thc/THC/PE_Cooling_Management/FUN_05.01.01_Thermal_Managemant_Mode_Determination/PECoolingMode ==
  VTHC_ServiceMode_flg : Inport
  VTHC_ChargingMode_flg : Inport  Port=2
  VTHC_CoolingMode_flg : Inport  Port=3
  VTHC_AfterrunningMode_flg : Inport  Port=4
  Constant12 : Constant  Value=ENUM_ACCMODE_COOLING  SampleTime=-1
  Constant15 : Constant  Value=ENUM_ACCMODE_OFF  SampleTime=-1
  Constant2 : Constant  Value=ENUM_ACCMODE_CHARGING  SampleTime=-1
  Constant3 : Constant  Value=ENUM_ACCMODE_AFTERRUNNING  SampleTime=-1
  Constant7 : Constant  Value=ENUM_ACCMODE_SERVICE  SampleTime=-1
  Switch{1..2,4..5} (4 alike) : Switch  Criteria=u2 ~= 0
  VTHC_PECoolingMode_enum : Outport  VectorParamsAs1DForOutWhenUnconnected=off
  wires:
  Constant15/1 -> Switch5/3
  Switch5/1 -> Switch1/3
  VTHC_AfterrunningMode_flg/1 -> Switch5/2
  Constant3/1 -> Switch5/1
  Switch4/1 -> VTHC_PECoolingMode_enum/1  "VTHC_PECoolingMode_enum"
  VTHC_CoolingMode_flg/1 -> Switch1/2
  Constant12/1 -> Switch1/1
  VTHC_ServiceMode_flg/1 -> Switch4/2
  Constant7/1 -> Switch4/1
  Switch2/1 -> Switch4/3
  VTHC_ChargingMode_flg/1 -> Switch2/2
  Switch1/1 -> Switch2/3
  Constant2/1 -> Switch2/1

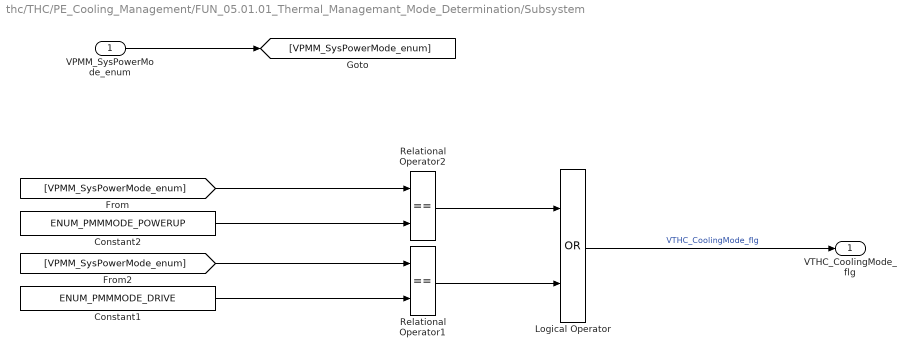
== system thc/THC/PE_Cooling_Management/FUN_05.01.01_Thermal_Managemant_Mode_Determination/Subsystem ==
  VPMM_SysPowerMode_enum : Inport
  Constant1 : Constant  Value=ENUM_PMMMODE_DRIVE  SampleTime=-1
  Constant2 : Constant  Value=ENUM_PMMMODE_POWERUP  SampleTime=-1
  Logical Operator : Logic  Operator=OR  AllPortsSameDT=off  OutDataTypeStr=boolean
  Relational Operator1 : RelationalOperator  Operator===  OutDataTypeStr=boolean  RndMeth=Nearest
  Relational Operator2 : RelationalOperator  Operator===  OutDataTypeStr=boolean  RndMeth=Nearest
  VTHC_CoolingMode_flg : Outport  VectorParamsAs1DForOutWhenUnconnected=off
  wires:
  Logical Operator/1 -> VTHC_CoolingMode_flg/1  "VTHC_CoolingMode_flg"
  Relational Operator1/1 -> Logical Operator/2
  Relational Operator2/1 -> Logical Operator/1
  VPMM_SysPowerMode_enum/1 -> [VPMM_SysPowerMode_enum]
  [VPMM_SysPowerMode_enum] -> Relational Operator2/1
  [VPMM_SysPowerMode_enum] -> Relational Operator1/1
  Constant1/1 -> Relational Operator1/2
  Constant2/1 -> Relational Operator2/2
